simulink model "test_matlab_system"  (Simulink 10.1)
settings: Solver=FixedStepAuto  StartTime=0.0  StopTime=Config.simulationTime  FixedStep=Config.tStep  RelTol=1e-3
InitFcn:
  | init
undefined symbols (not defined in the file or in its folder): Config, confVisualizer
settings Model: Creator=giuseppe  LastModifiedBy=giuseppe
settings DataIOCC: SaveFormat=Dataset  ReturnWorkspaceOutputs=on
settings OptimizationCC: LifeSpan=auto
settings DebuggingCC: UnderspecifiedInitializationDetection=Simplified  MergeDetectMultiDrivingBlocksExec=error  SFUnexpectedBacktrackingDiag=error  SFNoUnconditionalDefaultTransitionDiag=error  SFExecutionAtInitializationDiag=warning  ArithmeticOperatorsInVariantConditions=error
settings HardwareCC: ProdBitPerPointer=64  ProdBitPerSizeT=64  ProdBitPerPtrDiffT=64  ProdLargestAtomicFloat=Float  ProdIntDivRoundTo=Zero  ProdEndianess=LittleEndian  ProdWordSize=64  ProdHWDeviceType=Intel->x86-64 (Windows64)
settings ModelReferenceCC: PropagateSignalLabelsOutOfModel=on
settings SFSimCC: SimUseLocalCustomCode=on  CustomCodeUndefinedFunction=FilterOut
settings RTWCC: RTWUseLocalCustomCode=on
settings CodeAppCC: StateflowObjectComments=off
settings GRTTargetCC: TargetLangStandard=C99 (ISO)  CombineOutputUpdateFcns=on  GRTInterface=off
settings ConfigComp: CovMetricSettings=dwe  CovHtmlReporting=off  CovSaveCumulativeToWorkspaceVar=off  CovSaveSingleToWorkspaceVar=off  CovExternalEMLEnable=on

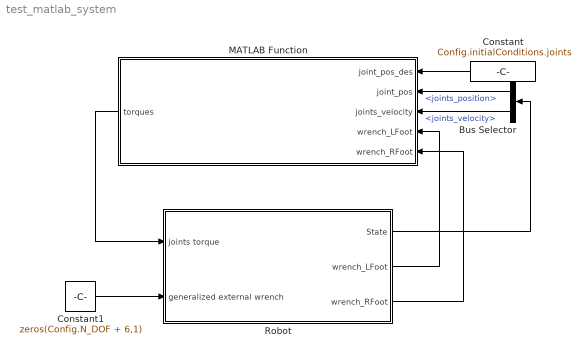
== system test_matlab_system ==
  Bus Selector : BusSelector  OutputSignals=joints_position,joints_velocity
  Constant : Constant  Value=Config.initialConditions.joints
  Constant1 : Constant  Value=zeros(Config.N_DOF + 6,1)
  MATLAB Function : MATLAB Function  TreatAsAtomicUnit=on
  Robot : Subsystem
  wires:
  Constant1/1 -> Robot/2(generalized external wrench)
  Bus Selector/1 -> MATLAB Function/2(joint_pos)  "<joints_position>"
  Bus Selector/2 -> MATLAB Function/3(joints_velocity)  "<joints_velocity>"
  Robot/1(State) -> Bus Selector/1
  Robot/2(wrench_LFoot) -> MATLAB Function/4(wrench_LFoot)
  Robot/3(wrench_RFoot) -> MATLAB Function/5(wrench_RFoot)
  Constant/1 -> MATLAB Function/1(joint_pos_des)
  MATLAB Function/1(torques) -> Robot/1(joints torque)

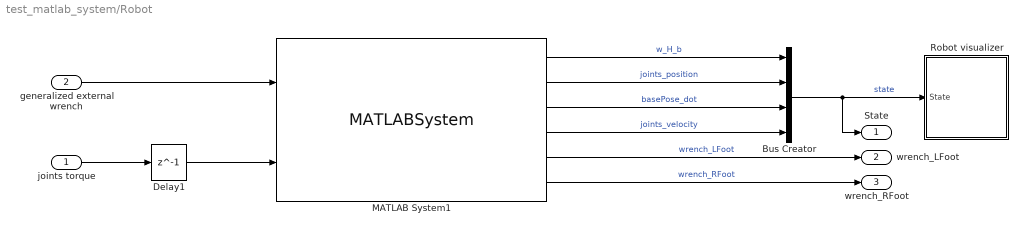
== system test_matlab_system/Robot ==
  joints torque : Inport
  generalized external wrench : Inport  Port=2
  Bus Creator : BusCreator  Inputs=4
  Delay1 : Delay  DelayLength=1  InitialCondition=zeros(23,1)
  MATLAB System1 : MATLABSystem  System=step_block  robot_config=robot_config  contact_config=contact_config  tStep=Config.tStep  SimulateUsing=Interpreted execution
      mask Type: step_block
      mask Display:
      | disp('step_block');
      | port_label('input',1,'generalized_ext_wrench');
      | port_label('input',2,'torque');
      | port_label('output',1,'w_H_b');
      | port_label('output',2,'s');
      | port_label('output',3,'base_pose_dot');
      | port_label('output',4,'s_dot');
      | port_label('output',5,'wrench_left_foot');
      | port_label('output',6,'wrench_right_foot');
  Robot visualizer : Subsystem  SystemSampleTime=confVisualizer.tStep
  State : Outport
  wrench_LFoot : Outport  Port=2
  wrench_RFoot : Outport  Port=3
  wires:
  Bus Creator/1 -> State/1, Robot visualizer/1(State)  "state"
  joints torque/1 -> Delay1/1
  MATLAB System1/5 -> wrench_LFoot/1  "wrench_LFoot"
  MATLAB System1/6 -> wrench_RFoot/1  "wrench_RFoot"
  MATLAB System1/1 -> Bus Creator/1  "w_H_b"
  MATLAB System1/2 -> Bus Creator/2  "joints_position"
  MATLAB System1/3 -> Bus Creator/3  "basePose_dot"
  MATLAB System1/4 -> Bus Creator/4  "joints_velocity"
  Delay1/1 -> MATLAB System1/2
  generalized external wrench/1 -> MATLAB System1/1

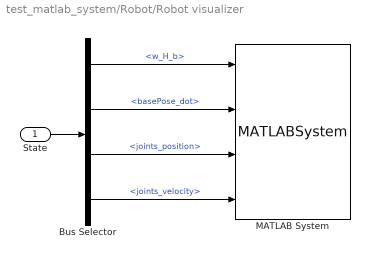
== system test_matlab_system/Robot/Robot visualizer ==
  State : Inport
  Bus Selector : BusSelector  OutputSignals=w_H_b,basePose_dot,joints_position,joints_velocity
  MATLAB System : MATLABSystem  System=Visualizer  config=confVisualizer  SimulateUsing=Interpreted execution
      mask Type: Visualizer
      mask Display:
      | disp(['Robot' char(10) 'Visualizer']);
      | port_label('input',1,'world_H_base');
      | port_label('input',2,'base_velocity');
      | port_label('input',3,'joints_positions');
      | port_label('input',4,'joints_velocity');
  wires:
  State/1 -> Bus Selector/1
  Bus Selector/1 -> MATLAB System/1  "<w_H_b>"
  Bus Selector/3 -> MATLAB System/3  "<joints_position>"
  Bus Selector/2 -> MATLAB System/2  "<basePose_dot>"
  Bus Selector/4 -> MATLAB System/4  "<joints_velocity>"

== matlab function MATLAB Function ==
  data: torques output double; joint_pos_des input double; joint_pos input double; joints_velocity input double; wrench_LFoot input double; wrench_RFoot input double
function torques = dummy_torque_control(joint_pos_des, joint_pos, joints_velocity, wrench_LFoot, wrench_RFoot)
    
    joints_pos_error = (joint_pos_des - joint_pos);
    
    KP = 0.1;
    KD = 2*sqrt(KP);
    
    torques = KP*(joints_pos_error) - KD*joints_velocity;
